simulink model "Lab_6_21"  (R2014a)
settings: Solver=ode45  StartTime=0.0  StopTime=5  RelTol=1e-3
values from neighbouring files (symbols this model uses):
  Be = Bm    (= 0.02)    [Lab_6_0.m]
  Je = Jo+Jm+(rm/r1)^2*J1+(rm/r1)^2*(r1/r2)^2*J2+(rm/r1)^2*mc*r1^2    (= 0.06001255625)    [Lab_6_0.m]
  K = [0,1]*(Pc^-1)*qa    [Lab_6_0.m]
  Kb = 0.060    (= 0.06)    [Lab_6_0.m]    (also in Project.m)
  Kt = 0.065    [Lab_6_0.m]    (also in Project.m)
  La = 0    [Lab_6_0.m]    (also in Project.m)
  pos = input('Enter desired steady-state position [mm]: ')/1000    [Lab_6_0.m]
  r1 = 0.008    [Lab_6_0.m]    (also in Project.m = input('Enter Pulley 1 Radius [m]: '))
  r2 = 0.008    [Lab_6_0.m]    (also in Project.m = input('Enter Pulley 2 Radius [m]: '))
  Ra = 1.5    [Lab_6_0.m]    (also in Project.m)
  rm = .005    (= 0.005)    [Lab_6_0.m]
undefined symbols (not defined in the file or in its folder): ramp
libraries: simulink x1
settings Model: Creator=muellerb  LastModifiedBy=muellerb

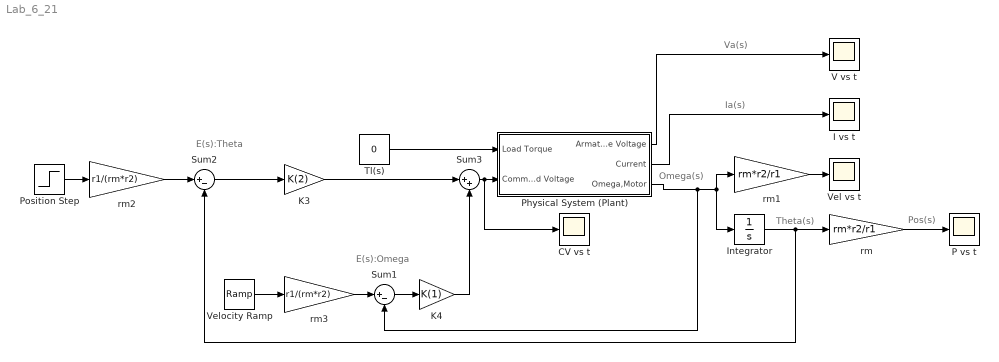
== system Lab_6_21 ==
  note: E(s):Theta
  note: Pos(s)
  note: Va(s)
  note: Theta(s)
  note: Omega(s)
  note: Ia(s)
  note: E(s):Omega
  CV vs t : Scope
      settings: SaveName=ScopeData4
  I vs t : Scope
      settings: SaveName=Current
  Integrator : Integrator
  K3 : Gain  Gain=K(2)
  K4 : Gain  Gain=K(1)
  P vs t : Scope
      settings: SaveName=Position
  Physical System (Plant) : Subsystem
  Position Step : Step  Time=0  After=pos  SampleTime=0
  Sum1 : Sum  Inputs=|+-
  Sum2 : Sum  Inputs=|+-
  Sum3 : Sum  Inputs=|++
  Tl(s) : Constant  Value=0
  V vs t : Scope
      settings: SaveName=Voltage
  Vel vs t : Scope
      settings: SaveName=ScopeData3
  Velocity Ramp : simulink/Sources/Ramp  slope=1  start=0  X0=ramp
  rm : Gain  Gain=rm*r2/r1
  rm1 : Gain  Gain=rm*r2/r1
  rm2 : Gain  Gain=r1/(rm*r2)
  rm3 : Gain  Gain=r1/(rm*r2)
  wires:
  rm/1 -> P vs t/1
  Integrator/1 -> Sum2/2, rm/1
  rm1/1 -> Vel vs t/1
  Position Step/1 -> rm2/1
  rm2/1 -> Sum2/1
  Velocity Ramp/1 -> rm3/1
  Sum2/1 -> K3/1
  Physical System (Plant)/3(Omega,Motor) -> Sum1/2, rm1/1, Integrator/1
  Tl(s)/1 -> Physical System (Plant)/1(Load Torque)
  Sum3/1 -> CV vs t/1, Physical System (Plant)/2(Command Voltage)
  Physical System (Plant)/1(Armature Voltage) -> V vs t/1
  Physical System (Plant)/2(Current) -> I vs t/1
  Sum1/1 -> K4/1
  K3/1 -> Sum3/1
  K4/1 -> Sum3/2
  rm3/1 -> Sum1/1

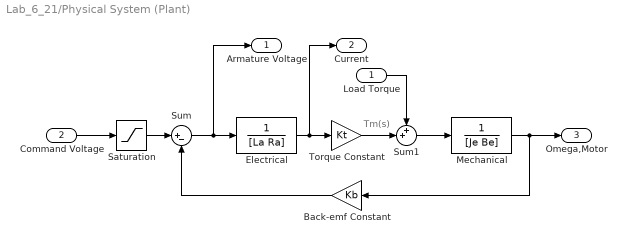
== system Lab_6_21/Physical System (Plant) ==
  note: Tm(s)
  Load Torque : Inport
  Command Voltage : Inport  Port=2
  Back-emf Constant : Gain  Gain=Kb
  Electrical : TransferFcn  Denominator=[La Ra]
  Mechanical : TransferFcn  Denominator=[Je Be]
  Saturation : Saturate  UpperLimit=24  LowerLimit=-24
  Sum : Sum  Inputs=|+-
  Sum1 : Sum  Inputs=++|
  Torque Constant : Gain  Gain=Kt
  Armature Voltage : Outport
  Current : Outport  Port=2
  Omega,Motor : Outport  Port=3
  wires:
  Sum/1 -> Armature Voltage/1, Electrical/1
  Electrical/1 -> Current/1, Torque Constant/1
  Sum1/1 -> Mechanical/1
  Back-emf Constant/1 -> Sum/2
  Torque Constant/1 -> Sum1/2
  Load Torque/1 -> Sum1/1
  Mechanical/1 -> Back-emf Constant/1, Omega,Motor/1
  Command Voltage/1 -> Saturation/1
  Saturation/1 -> Sum/1
